simulink model "DefaultCode2012_Edit"  (Simulink 7.9)
settings: Solver=ode45  StartTime=0.0  StopTime=inf  RelTol=1e-3
PreLoadFcn:
  | create_sim_variant
InitFcn:
  | create_sim_variant
libraries: vexBEST_lib x26, simulink x2
CloseFcn:
  | clear GAMEPAD_INP_SIM GAMEPAD_INP_RTW IS_GINP_SIM
settings Model: Creator=shiremat  LastModifiedBy=shiremat
settings OptimizationCC: OptimizeModelRefInitCode=on  LifeSpan=1
settings DebuggingCC: SolverPrmCheckMsg=none  FcnCallInpInsideContextMsg=Use local settings
settings RTWCC: SystemTargetFile=vex_ert.tlc  GenCodeOnly=on  GenerateMakefile=off  TemplateMakefile=none  Description=Embedded Target for easyC IDE  ProcessScript=vex_ert_make_rtw_hook
settings CodeAppCC: IgnoreCustomStorageClasses=off
settings ERTTargetCC: CodeReplacementLibrary=ANSI_C  MultiwordLength=2048  ExtModeMexFile=noextcomm  ERTCustomFileTemplate=example_file_process.tlc  ConvertIfToSwitch=off  SuppressUnreachableDefaultCases=off

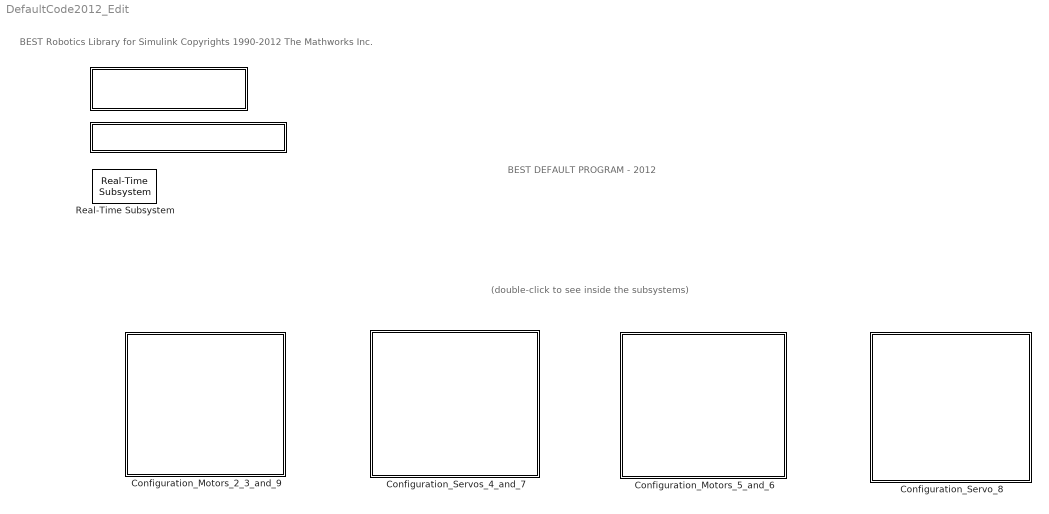
== system DefaultCode2012_Edit ==
  note: BEST Robotics Library for Simulink
      | Copyrights 1990-2012 The Mathworks Inc.
  note: (double-click to see inside the subsystems)
  note: BEST DEFAULT PROGRAM - 2012
  " " : Subsystem
      settings: OpenFcn=build_model_script  PreDeleteFcn="errordlg('Please do not delete the \"Generate Code\" block. Try Undo or Ctrl+Z to retrieve the block.','Error');"
      mask Display:
      | %image(imread('CodeGenButton.jpg'));
      | disp('Double-click to Generate Code')
  "  " : Subsystem
      settings: OpenFcn=vexBEST_lib  PreDeleteFcn="errordlg('Please do not delete the \"Generate Code\" block. Try Undo or Ctrl+Z to retrieve the block.','Error');"
      mask Display:
      | %image(imread('CodeGenButton.jpg'));
      | disp('Double-click to open BEST library')
  "Configuration_Motors_2_3_and_9 " : Subsystem
  Configuration_Motors_5_and_6 : Subsystem
  Configuration_Servo_8 : Subsystem
  "Configuration_Servos_4_and_7 " : Subsystem
  Real-Time Subsystem : vexBEST_lib/Utilities/Real-Time Subsystem  x=1

== system DefaultCode2012_Edit/  ==

== system DefaultCode2012_Edit/   ==

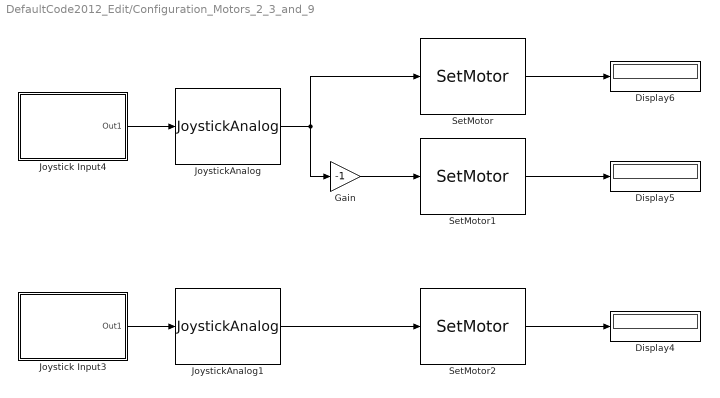
== system DefaultCode2012_Edit/Configuration_Motors_2_3_and_9  ==
  Display4 : Display
  Display5 : Display
  Display6 : Display
  Gain : Gain  Gain=-1
  Joystick Input3 : Subsystem
      settings: CopyFcn=set_param(gcb, 'LinkStatus', 'none') ;
      settings: NameChangeFcn=|
      | a=get_param(gcb, 'Blocks');
      | if strncmp(a{2}, 'Slider Gain', 6)
      | set_param([gcb, '/Slider Gain'], 'Name', get_param(gcb, 'Name'));
      | else
      | set_param([gcb, '/', a{2}], 'Name', get_param(gcb, 'Name'));
      | end
      settings: OpenFcn=|
      | try
      | set_param(gcb, 'LinkStatus', 'none') ;
      | a= get_param(gcb, 'Blocks');
      | open_system([gcb,'/',a{2}]);
      | close_system(gcs);
      | catch exception
      | errordlg('Add the block to a model to open and explore it.');
      | end
      mask Type: Joystick Input
      mask Description:
      | This is a source block that outputs values in the range -127 and 127.
      | The output value can be tuned using the slider control.
      mask Help:
      | This is a source block that outputs values in the range -127 and 127.
      | The output value can be tuned using the slider control.
      mask Display: image(imread('joystickanalogs.png'));
  Joystick Input4 : Subsystem
      settings: CopyFcn=set_param(gcb, 'LinkStatus', 'none') ;
      settings: NameChangeFcn=|
      | a=get_param(gcb, 'Blocks');
      | if strncmp(a{2}, 'Slider Gain', 6)
      | set_param([gcb, '/Slider Gain'], 'Name', get_param(gcb, 'Name'));
      | else
      | set_param([gcb, '/', a{2}], 'Name', get_param(gcb, 'Name'));
      | end
      settings: OpenFcn=|
      | try
      | set_param(gcb, 'LinkStatus', 'none') ;
      | a= get_param(gcb, 'Blocks');
      | open_system([gcb,'/',a{2}]);
      | close_system(gcs);
      | catch exception
      | errordlg('Add the block to a model to open and explore it.');
      | end
      mask Type: Joystick Input
      mask Description:
      | This is a source block that outputs values in the range -127 and 127.
      | The output value can be tuned using the slider control.
      mask Help:
      | This is a source block that outputs values in the range -127 and 127.
      | The output value can be tuned using the slider control.
      mask Display: image(imread('joystickanalogs.png'));
  JoystickAnalog : vexBEST_lib/JoystickAnalog  joystick=1  chan=3
  JoystickAnalog1 : vexBEST_lib/JoystickAnalog  joystick=1  chan=4
  SetMotor : vexBEST_lib/SetMotor  motor=2  scaleFactor=1/13.5
  SetMotor1 : vexBEST_lib/SetMotor  motor=9  scaleFactor=1/13.5
  SetMotor2 : vexBEST_lib/SetMotor  motor=3  scaleFactor=1/13.5
  wires:
  Gain/1 -> SetMotor1/1
  JoystickAnalog/1 -> SetMotor/1, Gain/1
  JoystickAnalog1/1 -> SetMotor2/1
  Joystick Input3/1(Out1) -> JoystickAnalog1/1
  Joystick Input4/1(Out1) -> JoystickAnalog/1
  SetMotor/1 -> Display6/1
  SetMotor1/1 -> Display5/1
  SetMotor2/1 -> Display4/1

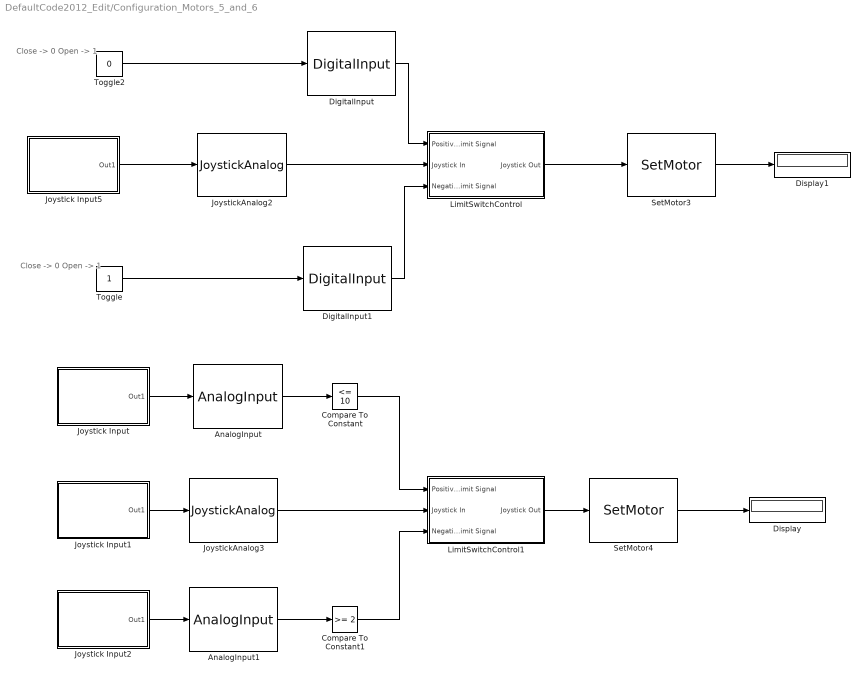
== system DefaultCode2012_Edit/Configuration_Motors_5_and_6 ==
  note: Close -> 0
      | Open -> 1
  note: Close -> 0
      | Open -> 1
  AnalogInput : vexBEST_lib/AnalogInput  inChan=1
  AnalogInput1 : vexBEST_lib/AnalogInput  inChan=1
  Compare To Constant : simulink/Logic and Bit Operations/Compare To Constant  relop=<=  const=10  OutDataTypeStr=boolean
  Compare To Constant1 : simulink/Logic and Bit Operations/Compare To Constant  relop=>=  const=2  OutDataTypeStr=boolean
  DigitalInput : vexBEST_lib/DigitalInput  inChan=1
  DigitalInput1 : vexBEST_lib/DigitalInput  inChan=2
  Display : Display
  Display1 : Display
  Joystick Input : Subsystem
      settings: CopyFcn=set_param(gcb, 'LinkStatus', 'none') ;
      settings: NameChangeFcn=|
      | a=get_param(gcb, 'Blocks');
      | if strncmp(a{2}, 'Slider Gain', 6)
      | set_param([gcb, '/Slider Gain'], 'Name', get_param(gcb, 'Name'));
      | else
      | set_param([gcb, '/', a{2}], 'Name', get_param(gcb, 'Name'));
      | end
      settings: OpenFcn=|
      | try
      | set_param(gcb, 'LinkStatus', 'none') ;
      | a= get_param(gcb, 'Blocks');
      | open_system([gcb,'/',a{2}]);
      | close_system(gcs);
      | catch exception
      | errordlg('Add the block to a model to open and explore it.');
      | end
      mask Type: Joystick Input
      mask Description:
      | This is a source block that outputs values in the range -127 and 127.
      | The output value can be tuned using the slider control.
      mask Help:
      | This is a source block that outputs values in the range -127 and 127.
      | The output value can be tuned using the slider control.
      mask Display: image(imread('joystickanalogs.png'));
  Joystick Input1 : Subsystem
      settings: CopyFcn=set_param(gcb, 'LinkStatus', 'none') ;
      settings: NameChangeFcn=|
      | a=get_param(gcb, 'Blocks');
      | if strncmp(a{2}, 'Slider Gain', 6)
      | set_param([gcb, '/Slider Gain'], 'Name', get_param(gcb, 'Name'));
      | else
      | set_param([gcb, '/', a{2}], 'Name', get_param(gcb, 'Name'));
      | end
      settings: OpenFcn=|
      | try
      | set_param(gcb, 'LinkStatus', 'none') ;
      | a= get_param(gcb, 'Blocks');
      | open_system([gcb,'/',a{2}]);
      | close_system(gcs);
      | catch exception
      | errordlg('Add the block to a model to open and explore it.');
      | end
      mask Type: Joystick Input
      mask Description:
      | This is a source block that outputs values in the range -127 and 127.
      | The output value can be tuned using the slider control.
      mask Help:
      | This is a source block that outputs values in the range -127 and 127.
      | The output value can be tuned using the slider control.
      mask Display: image(imread('joystickanalogs.png'));
  Joystick Input2 : Subsystem
      settings: CopyFcn=set_param(gcb, 'LinkStatus', 'none') ;
      settings: NameChangeFcn=|
      | a=get_param(gcb, 'Blocks');
      | if strncmp(a{2}, 'Slider Gain', 6)
      | set_param([gcb, '/Slider Gain'], 'Name', get_param(gcb, 'Name'));
      | else
      | set_param([gcb, '/', a{2}], 'Name', get_param(gcb, 'Name'));
      | end
      settings: OpenFcn=|
      | try
      | set_param(gcb, 'LinkStatus', 'none') ;
      | a= get_param(gcb, 'Blocks');
      | open_system([gcb,'/',a{2}]);
      | close_system(gcs);
      | catch exception
      | errordlg('Add the block to a model to open and explore it.');
      | end
      mask Type: Joystick Input
      mask Description:
      | This is a source block that outputs values in the range -127 and 127.
      | The output value can be tuned using the slider control.
      mask Help:
      | This is a source block that outputs values in the range -127 and 127.
      | The output value can be tuned using the slider control.
      mask Display: image(imread('joystickanalogs.png'));
  Joystick Input5 : Subsystem
      settings: CopyFcn=set_param(gcb, 'LinkStatus', 'none') ;
      settings: NameChangeFcn=|
      | a=get_param(gcb, 'Blocks');
      | if strncmp(a{2}, 'Slider Gain', 6)
      | set_param([gcb, '/Slider Gain'], 'Name', get_param(gcb, 'Name'));
      | else
      | set_param([gcb, '/', a{2}], 'Name', get_param(gcb, 'Name'));
      | end
      settings: OpenFcn=|
      | try
      | set_param(gcb, 'LinkStatus', 'none') ;
      | a= get_param(gcb, 'Blocks');
      | open_system([gcb,'/',a{2}]);
      | close_system(gcs);
      | catch exception
      | errordlg('Add the block to a model to open and explore it.');
      | end
      mask Type: Joystick Input
      mask Description:
      | This is a source block that outputs values in the range -127 and 127.
      | The output value can be tuned using the slider control.
      mask Help:
      | This is a source block that outputs values in the range -127 and 127.
      | The output value can be tuned using the slider control.
      mask Display: image(imread('joystickanalogs.png'));
  JoystickAnalog2 : vexBEST_lib/JoystickAnalog  joystick=1  chan=1
  JoystickAnalog3 : vexBEST_lib/JoystickAnalog  joystick=1  chan=2
  LimitSwitchControl : Subsystem
      mask Type: Limit Switch Control
      mask Description:
      | Connect Digital Input switches and a Joystick Analog signal to limit the range of motion of a motor.  The physical switches should be installed such that they are depressed when the actuated components are at their extremes of motion.
      | 
      | This module will prevent motion in the corresponding direction if a digital switch is depressed.
      mask Help:
      | Connect Digital Input switches and a Joystick Analog signal to limit the range of motion of a motor.  The physical switches should be installed such that they are depressed when the actuated components are at their extremes of motion.
      | 
      | This module will prevent motion in the corresponding direction if a digital switch is depressed.
  LimitSwitchControl1 : Subsystem
      mask Type: Limit Switch Control
      mask Description:
      | Connect Digital Input switches and a Joystick Analog signal to limit the range of motion of a motor.  The physical switches should be installed such that they are depressed when the actuated components are at their extremes of motion.
      | 
      | This module will prevent motion in the corresponding direction if a digital switch is depressed.
      mask Help:
      | Connect Digital Input switches and a Joystick Analog signal to limit the range of motion of a motor.  The physical switches should be installed such that they are depressed when the actuated components are at their extremes of motion.
      | 
      | This module will prevent motion in the corresponding direction if a digital switch is depressed.
  SetMotor3 : vexBEST_lib/SetMotor  motor=5  scaleFactor=1/13.5
  SetMotor4 : vexBEST_lib/SetMotor  motor=6  scaleFactor=1/13.5
  Toggle : Constant
      settings: OpenFcn=|
      | if strcmp('0',get_param(gcb, 'Value'))                        set_param(gcb, 'Value', '1');
      | else
      |             set_param(gcb, 'Value', '0');
      | end
  Toggle2 : Constant  Value=0
      settings: OpenFcn=|
      | if strcmp('0',get_param(gcb, 'Value'))                        set_param(gcb, 'Value', '1');
      | else
      |             set_param(gcb, 'Value', '0');
      | end
  wires:
  JoystickAnalog2/1 -> LimitSwitchControl/2(Joystick In)
  DigitalInput/1 -> LimitSwitchControl/1(Positive Limit Signal)
  DigitalInput1/1 -> LimitSwitchControl/3(Negative Limit Signal)
  LimitSwitchControl1/1(Joystick Out) -> SetMotor4/1
  JoystickAnalog3/1 -> LimitSwitchControl1/2(Joystick In)
  Compare To Constant/1 -> LimitSwitchControl1/1(Positive Limit Signal)
  Compare To Constant1/1 -> LimitSwitchControl1/3(Negative Limit Signal)
  AnalogInput/1 -> Compare To Constant/1
  AnalogInput1/1 -> Compare To Constant1/1
  Joystick Input/1(Out1) -> AnalogInput/1
  Joystick Input1/1(Out1) -> JoystickAnalog3/1
  Joystick Input2/1(Out1) -> AnalogInput1/1
  SetMotor4/1 -> Display/1
  SetMotor3/1 -> Display1/1
  Toggle/1 -> DigitalInput1/1
  Joystick Input5/1(Out1) -> JoystickAnalog2/1
  Toggle2/1 -> DigitalInput/1
  LimitSwitchControl/1(Joystick Out) -> SetMotor3/1

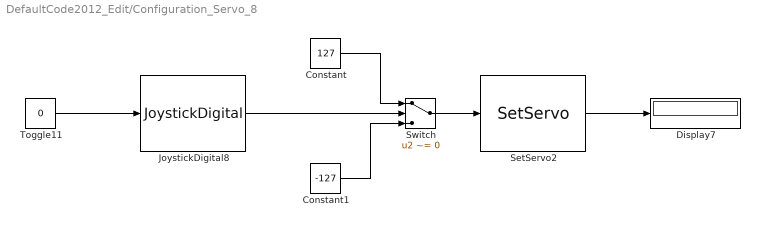
== system DefaultCode2012_Edit/Configuration_Servo_8 ==
  Constant : Constant  Value=127
  Constant1 : Constant  Value=-127
  Display7 : Display
  JoystickDigital8 : vexBEST_lib/JoystickDigital  joystick=1  chan=6  button56=Up  button78=Left
  SetServo2 : vexBEST_lib/SetServo  motor=8  scaleFactor=90/127
  Switch : Switch  Criteria=u2 ~= 0
  Toggle11 : Constant  Value=0
      settings: OpenFcn=|
      | if strcmp('0',get_param(gcb, 'Value'))                        set_param(gcb, 'Value', '1');
      | else
      |             set_param(gcb, 'Value', '0');
      | end
  wires:
  SetServo2/1 -> Display7/1
  Toggle11/1 -> JoystickDigital8/1
  Switch/1 -> SetServo2/1
  Constant/1 -> Switch/1
  JoystickDigital8/1 -> Switch/2
  Constant1/1 -> Switch/3

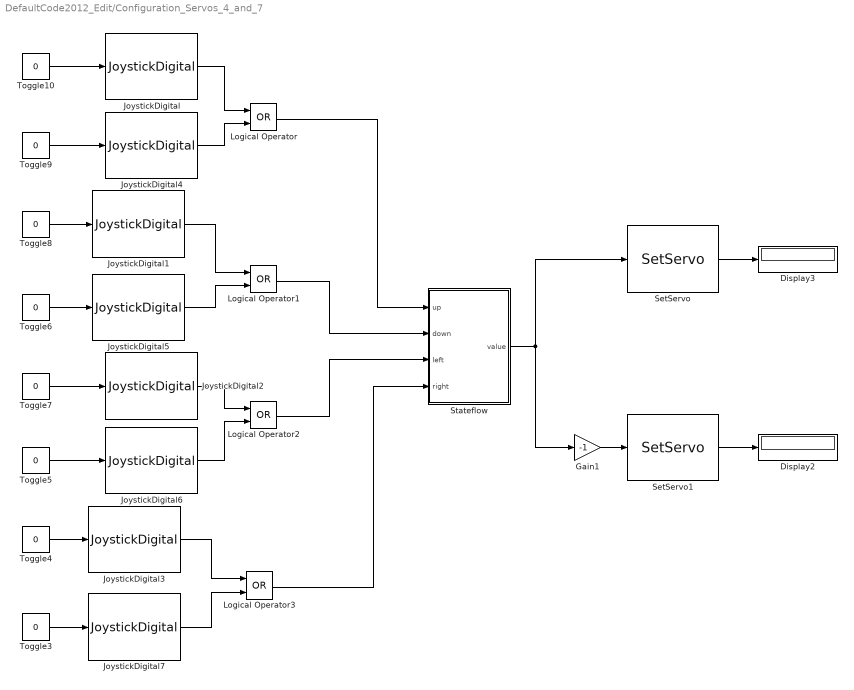
== system DefaultCode2012_Edit/Configuration_Servos_4_and_7  ==
  Display2 : Display
  Display3 : Display
  Gain1 : Gain  Gain=-1
  JoystickDigital : vexBEST_lib/JoystickDigital  joystick=1  chan=7  button56=Down  button78=Up
  JoystickDigital1 : vexBEST_lib/JoystickDigital  joystick=1  chan=7  button56=Down  button78=Down
  JoystickDigital2 : vexBEST_lib/JoystickDigital  joystick=1  chan=7  button56=Down  button78=Left
  JoystickDigital3 : vexBEST_lib/JoystickDigital  joystick=1  chan=7  button56=Down  button78=Right
  JoystickDigital4 : vexBEST_lib/JoystickDigital  joystick=1  chan=8  button56=Down  button78=Up
  JoystickDigital5 : vexBEST_lib/JoystickDigital  joystick=1  chan=8  button56=Down  button78=Down
  JoystickDigital6 : vexBEST_lib/JoystickDigital  joystick=1  chan=8  button56=Down  button78=Left
  JoystickDigital7 : vexBEST_lib/JoystickDigital  joystick=1  chan=8  button56=Down  button78=Right
  Logical Operator{,1..3} (4 alike) : Logic  Operator=OR  AllPortsSameDT=off  OutDataTypeStr=boolean
  SetServo : vexBEST_lib/SetServo  motor=4  scaleFactor=90/127
  SetServo1 : vexBEST_lib/SetServo  motor=7  scaleFactor=90/127
  Stateflow : Stateflow chart  TreatAsAtomicUnit=on
      settings: CopyFcn=|
      | % delete the link so that this is editable
      | set_param(gcb, 'LinkStatus', 'none');
  Toggle{3..10} (8 alike) : Constant  Value=0
      settings: OpenFcn=|
      | if strcmp('0',get_param(gcb, 'Value'))                        set_param(gcb, 'Value', '1');
      | else
      |             set_param(gcb, 'Value', '0');
      | end
  wires:
  JoystickDigital/1 -> Logical Operator/1
  JoystickDigital4/1 -> Logical Operator/2
  JoystickDigital1/1 -> Logical Operator1/1
  JoystickDigital5/1 -> Logical Operator1/2
  JoystickDigital2/1 -> Logical Operator2/1
  JoystickDigital6/1 -> Logical Operator2/2
  JoystickDigital3/1 -> Logical Operator3/1
  JoystickDigital7/1 -> Logical Operator3/2
  Logical Operator/1 -> Stateflow/1(up)
  Logical Operator1/1 -> Stateflow/2(down)
  Logical Operator2/1 -> Stateflow/3(left)
  Logical Operator3/1 -> Stateflow/4(right)
  Stateflow/1(value) -> SetServo/1, Gain1/1
  Gain1/1 -> SetServo1/1
  Toggle3/1 -> JoystickDigital7/1
  Toggle4/1 -> JoystickDigital3/1
  Toggle5/1 -> JoystickDigital6/1
  Toggle6/1 -> JoystickDigital5/1
  Toggle7/1 -> JoystickDigital2/1
  Toggle8/1 -> JoystickDigital1/1
  Toggle9/1 -> JoystickDigital4/1
  Toggle10/1 -> JoystickDigital/1
  SetServo1/1 -> Display2/1
  SetServo/1 -> Display3/1

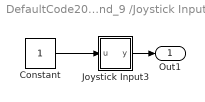
== system DefaultCode2012_Edit/Configuration_Motors_2_3_and_9 /Joystick Input3 ==
  Constant : Constant
  Joystick Input3 : Subsystem  LoadFcn=slideg Load  StartFcn=slideg StartFcn  StopFcn=slideg StopFcn  mask(Slider Gain){low=-127, gain=0, high=127}
      settings: CopyFcn=slideg Copy  DeleteFcn=slideg DeleteBlock  NameChangeFcn=slideg NameChange  OpenFcn=slideg Open  CloseFcn=slideg Close
      mask Display: disp(gain)
  Out1 : Outport
  wires:
  Constant/1 -> Joystick Input3/1(u)
  Joystick Input3/1(y) -> Out1/1

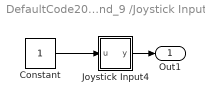
== system DefaultCode2012_Edit/Configuration_Motors_2_3_and_9 /Joystick Input4 ==
  Constant : Constant
  Joystick Input4 : Subsystem  LoadFcn=slideg Load  StartFcn=slideg StartFcn  StopFcn=slideg StopFcn  mask(Slider Gain){low=-127, gain=0, high=127}
      settings: CopyFcn=slideg Copy  DeleteFcn=slideg DeleteBlock  NameChangeFcn=slideg NameChange  OpenFcn=slideg Open  CloseFcn=slideg Close
      mask Display: disp(gain)
  Out1 : Outport
  wires:
  Joystick Input4/1(y) -> Out1/1
  Constant/1 -> Joystick Input4/1(u)

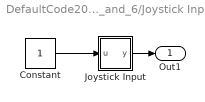
== system DefaultCode2012_Edit/Configuration_Motors_5_and_6/Joystick Input ==
  Constant : Constant
  Joystick Input : Subsystem  LoadFcn=slideg Load  StartFcn=slideg StartFcn  StopFcn=slideg StopFcn  mask(Slider Gain){low=-127, gain=10.16, high=127}
      settings: CopyFcn=slideg Copy  DeleteFcn=slideg DeleteBlock  NameChangeFcn=slideg NameChange  OpenFcn=slideg Open  CloseFcn=slideg Close
      mask Display: disp(gain)
  Out1 : Outport
  wires:
  Joystick Input/1(y) -> Out1/1
  Constant/1 -> Joystick Input/1(u)

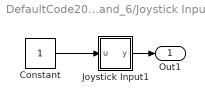
== system DefaultCode2012_Edit/Configuration_Motors_5_and_6/Joystick Input1 ==
  Constant : Constant
  Joystick Input1 : Subsystem  LoadFcn=slideg Load  StartFcn=slideg StartFcn  StopFcn=slideg StopFcn  mask(Slider Gain){low=-127, gain=-40.7805, high=127}
      settings: CopyFcn=slideg Copy  DeleteFcn=slideg DeleteBlock  NameChangeFcn=slideg NameChange  OpenFcn=slideg Open  CloseFcn=slideg Close
      mask Display: disp(gain)
  Out1 : Outport
  wires:
  Constant/1 -> Joystick Input1/1(u)
  Joystick Input1/1(y) -> Out1/1

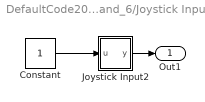
== system DefaultCode2012_Edit/Configuration_Motors_5_and_6/Joystick Input2 ==
  Constant : Constant
  Joystick Input2 : Subsystem  LoadFcn=slideg Load  StartFcn=slideg StartFcn  StopFcn=slideg StopFcn  mask(Slider Gain){low=-127, gain=-1.54, high=127}
      settings: CopyFcn=slideg Copy  DeleteFcn=slideg DeleteBlock  NameChangeFcn=slideg NameChange  OpenFcn=slideg Open  CloseFcn=slideg Close
      mask Display: disp(gain)
  Out1 : Outport
  wires:
  Joystick Input2/1(y) -> Out1/1
  Constant/1 -> Joystick Input2/1(u)

== system DefaultCode2012_Edit/Configuration_Motors_5_and_6/Joystick Input5 ==
  Constant : Constant
  Joystick Input5 : Subsystem  LoadFcn=slideg Load  StartFcn=slideg StartFcn  StopFcn=slideg StopFcn  mask(Slider Gain){low=-127, gain=-22.86, high=127}
      settings: CopyFcn=slideg Copy  DeleteFcn=slideg DeleteBlock  NameChangeFcn=slideg NameChange  OpenFcn=slideg Open  CloseFcn=slideg Close
      mask Display: disp(gain)
  Out1 : Outport
  wires:
  Constant/1 -> Joystick Input5/1(u)
  Joystick Input5/1(y) -> Out1/1

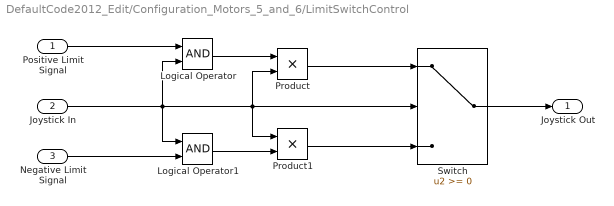
== system DefaultCode2012_Edit/Configuration_Motors_5_and_6/LimitSwitchControl ==
  Positive Limit Signal : Inport
  Joystick In : Inport  Port=2  OutDataTypeStr=double
  Negative Limit Signal : Inport  Port=3
  Logical Operator : Logic  AllPortsSameDT=off  OutDataTypeStr=boolean
  Logical Operator1 : Logic  AllPortsSameDT=off  OutDataTypeStr=boolean
  Product : Product  RndMeth=Zero
  Product1 : Product  RndMeth=Zero
  Switch : Switch
  Joystick Out : Outport
  wires:
  Product1/1 -> Switch/3
  Logical Operator1/1 -> Product1/2
  Product/1 -> Switch/1
  Logical Operator/1 -> Product/1
  Negative Limit Signal/1 -> Logical Operator1/2
  Positive Limit Signal/1 -> Logical Operator/1
  Joystick In/1 -> Product1/1, Product/2, Switch/2, Logical Operator1/1, Logical Operator/2
  Switch/1 -> Joystick Out/1

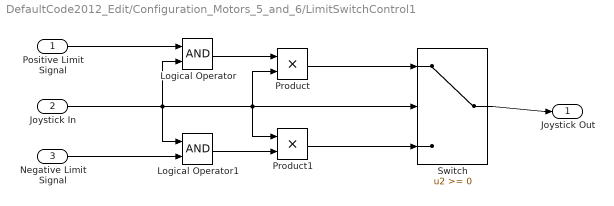
== system DefaultCode2012_Edit/Configuration_Motors_5_and_6/LimitSwitchControl1 ==
  Positive Limit Signal : Inport
  Joystick In : Inport  Port=2  OutDataTypeStr=double
  Negative Limit Signal : Inport  Port=3
  Logical Operator : Logic  AllPortsSameDT=off  OutDataTypeStr=boolean
  Logical Operator1 : Logic  AllPortsSameDT=off  OutDataTypeStr=boolean
  Product : Product  RndMeth=Zero
  Product1 : Product  RndMeth=Zero
  Switch : Switch
  Joystick Out : Outport
  wires:
  Product1/1 -> Switch/3
  Logical Operator1/1 -> Product1/2
  Product/1 -> Switch/1
  Logical Operator/1 -> Product/1
  Negative Limit Signal/1 -> Logical Operator1/2
  Positive Limit Signal/1 -> Logical Operator/1
  Joystick In/1 -> Product1/1, Product/2, Switch/2, Logical Operator1/1, Logical Operator/2
  Switch/1 -> Joystick Out/1

== system DefaultCode2012_Edit/Configuration_Motors_2_3_and_9 /Joystick Input3/Joystick Input3 ==
  u : Inport
  Slider Gain : Gain  Gain=gain  SaturateOnIntegerOverflow=on  OutDataTypeStr=Inherit: Same as input  ParamDataTypeStr=Inherit: Same as input
  y : Outport
  wires:
  Slider Gain/1 -> y/1
  u/1 -> Slider Gain/1

== system DefaultCode2012_Edit/Configuration_Motors_2_3_and_9 /Joystick Input4/Joystick Input4 ==
  u : Inport
  Slider Gain : Gain  Gain=gain  SaturateOnIntegerOverflow=on  OutDataTypeStr=Inherit: Same as input  ParamDataTypeStr=Inherit: Same as input
  y : Outport
  wires:
  u/1 -> Slider Gain/1
  Slider Gain/1 -> y/1

== system DefaultCode2012_Edit/Configuration_Motors_5_and_6/Joystick Input/Joystick Input ==
  u : Inport
  Slider Gain : Gain  Gain=gain  SaturateOnIntegerOverflow=on  OutDataTypeStr=Inherit: Same as input  ParamDataTypeStr=Inherit: Same as input
  y : Outport
  wires:
  u/1 -> Slider Gain/1
  Slider Gain/1 -> y/1

== system DefaultCode2012_Edit/Configuration_Motors_5_and_6/Joystick Input1/Joystick Input1 ==
  u : Inport
  Slider Gain : Gain  Gain=gain  SaturateOnIntegerOverflow=on  OutDataTypeStr=Inherit: Same as input  ParamDataTypeStr=Inherit: Same as input
  y : Outport
  wires:
  Slider Gain/1 -> y/1
  u/1 -> Slider Gain/1

== system DefaultCode2012_Edit/Configuration_Motors_5_and_6/Joystick Input2/Joystick Input2 ==
  u : Inport
  Slider Gain : Gain  Gain=gain  SaturateOnIntegerOverflow=on  OutDataTypeStr=Inherit: Same as input  ParamDataTypeStr=Inherit: Same as input
  y : Outport
  wires:
  u/1 -> Slider Gain/1
  Slider Gain/1 -> y/1

== system DefaultCode2012_Edit/Configuration_Motors_5_and_6/Joystick Input5/Joystick Input5 ==
  u : Inport
  Slider Gain : Gain  Gain=gain  SaturateOnIntegerOverflow=on  OutDataTypeStr=Inherit: Same as input  ParamDataTypeStr=Inherit: Same as input
  y : Outport
  wires:
  Slider Gain/1 -> y/1
  u/1 -> Slider Gain/1

== stateflow chart Configuration_Servos_4_and_7 /Stateflow ==
  state Idle
  (default) -> Idle : {value=-127}
  Idle -> Idle [order 1] : [up==1]{value=-127}
  Idle -> Idle [order 2] : [down==1]{value=-50}
  Idle -> Idle [order 3] : [left==1]{value=50}
  Idle -> Idle [order 4] : [right==1]{value=127}
  data: up input double; down input double; left input double; right input double; value output double
